simulink model "cl"  (Simulink 6.3)
settings: Solver=ode1  StartTime=0.0  StopTime=tsim_max  FixedStep=delt  RelTol=1e-3
values from neighbouring files (symbols this model uses):
  g = lp(i,1)    [gpm.m]
undefined symbols (not defined in the file or in its folder): Aac_trac, Asn, att1_step_cmd, att2_step_cmd, att3_step_cmd, att_type, Bac_trac, Bsn, c_att, c_rate, c_vel, ca_rate, ca_vel, Cac_trac, cbinv_rate, cbinv_vel, command_time, cosa, Cpos, ctht, Cvelpos, Dac_trac, delt, fb_att, fc_att, fc_pos, fc_rate, fc_vel, ff_att, fi_att, fi_pos, fi_rate, fi_vel, gthrot_step_cmd, ideal_d_actuator, ideal_engine_actuator, integ_d_a, integ_d_b, integ_d_c, integ_d_d, integ_engine_a, integ_engine_b, integ_engine_c, integ_engine_d, integ_gust_a, integ_gust_b, integ_gust_c, integ_gust_d, integ_MACH_att_a, integ_MACH_att_b, integ_MACH_att_c, integ_MACH_att_d, integ_MACH_att_ff_a, integ_MACH_att_ff_b, integ_MACH_att_ff_c, integ_MACH_att_ff_d, integ_MACH_pos_a, integ_MACH_pos_b, integ_MACH_pos_c, integ_MACH_pos_d ... (+53)
libraries: simulink x22
settings Model: LastModifiedBy=E704491  BufferReuse=off
settings DataIOCC: InitialState=[]  LoadInitialState=on
settings OptimizationCC: InlineParams=on  BufferReuse=off
settings DebuggingCC: AlgebraicLoopMsg=none

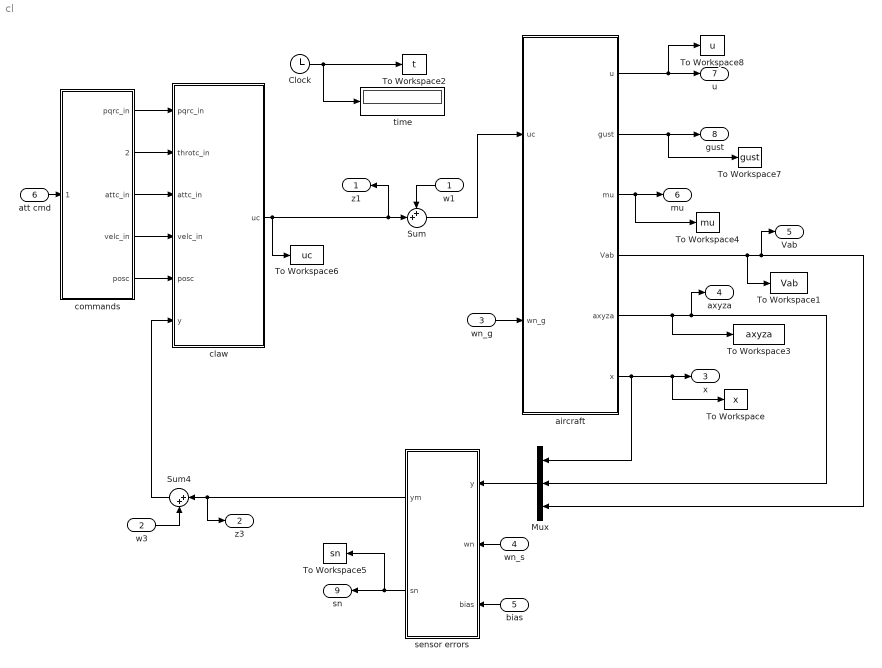
== system cl ==
  w1 : Inport  Orientation=left  PortDimensions=num_u
  w3 : Inport  Port=2  PortDimensions=num_y
  wn_g : Inport  Port=3  PortDimensions=3
  wn_s : Inport  Orientation=left  Port=4  PortDimensions=num_y
  bias : Inport  Orientation=left  Port=5  PortDimensions=num_y
  att cmd : Inport  Port=6
  Clock : Clock
      settings: Decimation=10
  Mux : Mux  Orientation=left  Inputs=3
  Sum : Sum  Inputs=++|
  Sum4 : Sum  Orientation=left  Inputs=|++
  To Workspace : ToWorkspace  VariableName=x  SampleTime=-1  SaveFormat=Array
  To Workspace1 : ToWorkspace  VariableName=Vab  SampleTime=-1  SaveFormat=Array
  To Workspace2 : ToWorkspace  VariableName=t  SampleTime=-1  SaveFormat=Array
  To Workspace3 : ToWorkspace  VariableName=axyza  SampleTime=-1  SaveFormat=Array
  To Workspace4 : ToWorkspace  VariableName=mu  SampleTime=-1  SaveFormat=Array
  To Workspace5 : ToWorkspace  VariableName=sn  SampleTime=-1  SaveFormat=Array
  To Workspace6 : ToWorkspace  VariableName=uc  SampleTime=-1  SaveFormat=Array
  To Workspace7 : ToWorkspace  VariableName=gust  SampleTime=-1  SaveFormat=Array
  To Workspace8 : ToWorkspace  VariableName=u  SampleTime=-1  SaveFormat=Array
  aircraft : Subsystem
  claw : Subsystem
  commands : Subsystem
  sensor errors : Subsystem  Orientation=left
  time : Display
  z1 : Outport  Orientation=left
  z3 : Outport  Port=2
  x : Outport  Port=3
  axyza : Outport  Port=4
  Vab : Outport  Port=5
  mu : Outport  Port=6
  u : Outport  Port=7
  gust : Outport  Port=8
  sn : Outport  Orientation=left  Port=9
  wires:
  claw/1(uc) -> Sum/2, z1/1, To Workspace6/1
  Clock/1 -> To Workspace2/1, time/1
  wn_s/1 -> sensor errors/2(wn)
  sensor errors/2(sn) -> sn/1, To Workspace5/1
  bias/1 -> sensor errors/3(bias)
  w1/1 -> Sum/1
  sensor errors/1(ym) -> Sum4/1, z3/1
  Sum4/1 -> claw/6(y)
  w3/1 -> Sum4/2
  aircraft/6(x) -> x/1, To Workspace/1, Mux/1
  aircraft/1(u) -> u/1, To Workspace8/1
  aircraft/4(Vab) -> To Workspace1/1, Vab/1, Mux/3
  Sum/1 -> aircraft/1(uc)
  wn_g/1 -> aircraft/2(wn_g)
  aircraft/2(gust) -> gust/1, To Workspace7/1
  commands/4(velc_in) -> claw/4(velc_in)
  aircraft/5(axyza) -> axyza/1, Mux/2, To Workspace3/1
  commands/5(posc) -> claw/5(posc)
  commands/2(throtc_in) -> claw/2(throtc_in)
  commands/3(attc_in) -> claw/3(attc_in)
  att cmd/1 -> commands/1(att cmd)
  Mux/1 -> sensor errors/1(y)
  aircraft/3(mu) -> mu/1, To Workspace4/1
  commands/1(pqrc_in) -> claw/1(pqrc_in)

== system cl/aircraft ==
  uc : Inport
  wn_g : Inport  Port=2
  actuators : Subsystem
  aircraft : Subsystem
  gust model : Subsystem
  u : Outport
  gust : Outport  Port=2
  mu : Outport  Port=3
  Vab : Outport  Port=4
  axyza : Outport  Port=5
  x : Outport  Port=6
  wires:
  aircraft/1(x) -> x/1
  aircraft/3(Vab) -> Vab/1
  wn_g/1 -> gust model/1(wn)
  gust model/1(gust) -> aircraft/2(gust), gust/1
  uc/1 -> actuators/1(uc)
  actuators/1(u) -> aircraft/1(u), u/1
  aircraft/2(axyza) -> axyza/1
  aircraft/4(mu) -> mu/1

== system cl/claw ==
  pqrc_in : Inport
  throtc_in : Inport  Port=2
  attc_in : Inport  Port=3
  velc_in : Inport  Port=4
  posc : Inport  Port=5
  y : Inport  Port=6
  MACH : Subsystem
  Mux : Mux  Inputs=2
  Mux1 : Mux  Inputs=5
  uc : Outport
  wires:
  attc_in/1 -> Mux1/3
  velc_in/1 -> Mux1/4
  Mux1/1 -> MACH/1(cmd)
  posc/1 -> Mux1/5
  y/1 -> MACH/2(y)
  MACH/1(d cmd) -> Mux/1
  MACH/2(throttle cmd) -> Mux/2
  Mux/1 -> uc/1
  throtc_in/1 -> Mux1/2
  pqrc_in/1 -> Mux1/1

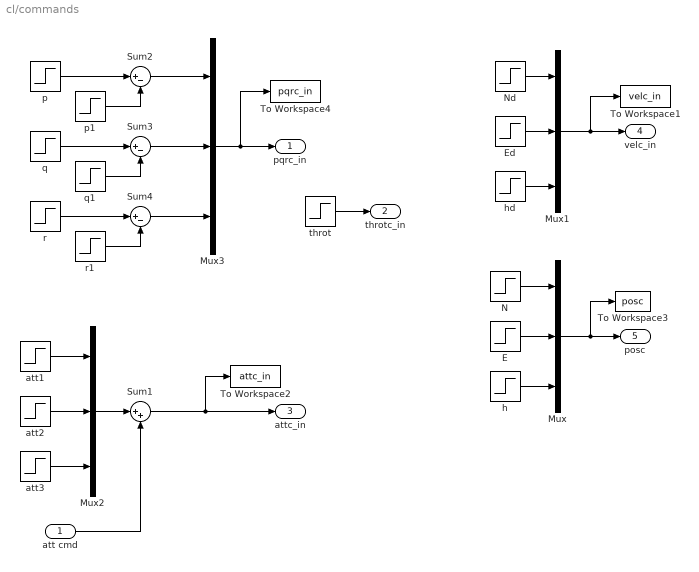
== system cl/commands ==
  att cmd : Inport  PortDimensions=3
  E : Step  Time=command_time  After=pos2_step_cmd  SampleTime=0
  Ed : Step  Time=command_time  After=vel2_step_cmd  SampleTime=0
  Mux{,1..3} (4 alike) : Mux  Inputs=3
  N : Step  Time=command_time  After=pos1_step_cmd  SampleTime=0
  Nd : Step  Time=command_time  After=vel1_step_cmd  SampleTime=0
  Sum1 : Sum  Inputs=|++
  Sum2 : Sum  Inputs=|+-
  Sum3 : Sum  Inputs=|+-
  Sum4 : Sum  Inputs=|+-
  To Workspace1 : ToWorkspace  VariableName=velc_in  SampleTime=-1  SaveFormat=Array
  To Workspace2 : ToWorkspace  VariableName=attc_in  SampleTime=-1  SaveFormat=Array
  To Workspace3 : ToWorkspace  VariableName=posc  SampleTime=-1  SaveFormat=Array
  To Workspace4 : ToWorkspace  VariableName=pqrc_in  SampleTime=-1  SaveFormat=Array
  att1 : Step  Time=command_time  After=att1_step_cmd  SampleTime=0
  att2 : Step  Time=command_time  After=att2_step_cmd  SampleTime=0
  att3 : Step  Time=command_time  After=att3_step_cmd  SampleTime=0
  h : Step  Time=command_time  After=pos3_step_cmd  SampleTime=0
  hd : Step  Time=command_time  After=vel3_step_cmd  SampleTime=0
  p : Step  Time=command_time  After=rate1_step_cmd  SampleTime=0
  p1 : Step  Time=command_time + pulse_width  After=rate1_step_cmd  SampleTime=0
  q : Step  Time=command_time  After=rate2_step_cmd  SampleTime=0
  q1 : Step  Time=command_time + pulse_width  After=rate2_step_cmd  SampleTime=0
  r : Step  Time=command_time  After=rate3_step_cmd  SampleTime=0
  r1 : Step  Time=command_time + pulse_width  After=rate3_step_cmd  SampleTime=0
  throt : Step  Time=command_time  After=gthrot_step_cmd  SampleTime=0
  pqrc_in : Outport
  throtc_in : Outport  Port=2
  attc_in : Outport  Port=3
  velc_in : Outport  Port=4
  posc : Outport  Port=5
  wires:
  h/1 -> Mux/3
  Nd/1 -> Mux1/1
  throt/1 -> throtc_in/1
  att2/1 -> Mux2/2
  att cmd/1 -> Sum1/2
  Mux/1 -> To Workspace3/1, posc/1
  Mux1/1 -> velc_in/1, To Workspace1/1
  att1/1 -> Mux2/1
  att3/1 -> Mux2/3
  Sum1/1 -> attc_in/1, To Workspace2/1
  Mux2/1 -> Sum1/1
  Mux3/1 -> pqrc_in/1, To Workspace4/1
  Sum2/1 -> Mux3/1
  p/1 -> Sum2/1
  Sum3/1 -> Mux3/2
  q/1 -> Sum3/1
  r/1 -> Sum4/1
  Sum4/1 -> Mux3/3
  p1/1 -> Sum2/2
  q1/1 -> Sum3/2
  r1/1 -> Sum4/2
  Ed/1 -> Mux1/2
  hd/1 -> Mux1/3
  N/1 -> Mux/1
  E/1 -> Mux/2

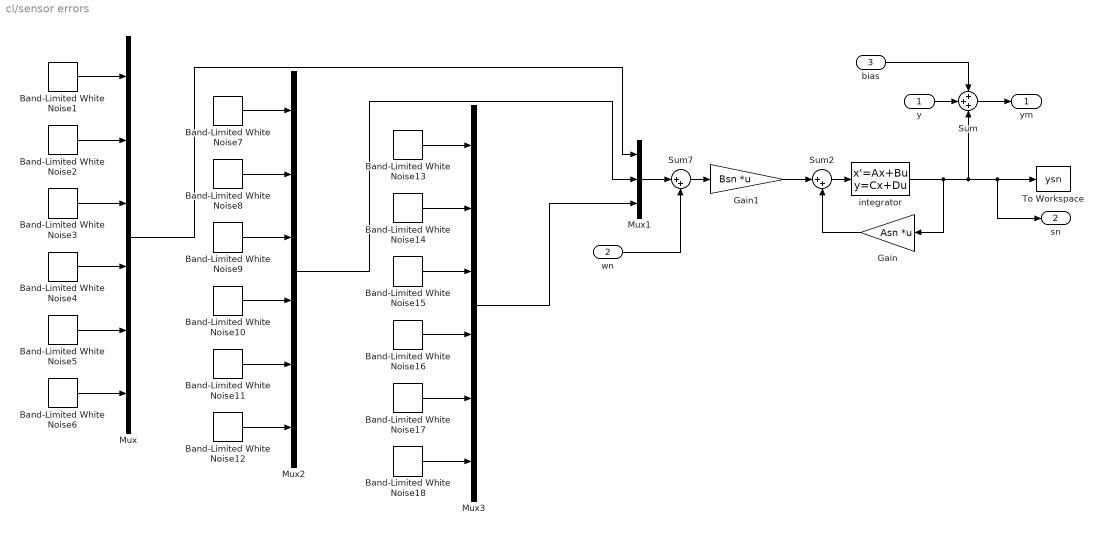
== system cl/sensor errors ==
  y : Inport
  wn : Inport  Port=2
  bias : Inport  Port=3
  Band-Limited White Noise1 : simulink/Sources/Band-Limited White Noise  Cov=1  Ts=delt  seed=sn_seed(1)
  Band-Limited White Noise10 : simulink/Sources/Band-Limited White Noise  Cov=1  Ts=delt  seed=sn_seed(10)
  Band-Limited White Noise11 : simulink/Sources/Band-Limited White Noise  Cov=1  Ts=delt  seed=sn_seed(11)
  Band-Limited White Noise12 : simulink/Sources/Band-Limited White Noise  Cov=1  Ts=delt  seed=sn_seed(12)
  Band-Limited White Noise13 : simulink/Sources/Band-Limited White Noise  Cov=1  Ts=delt  seed=sn_seed(13)
  Band-Limited White Noise14 : simulink/Sources/Band-Limited White Noise  Cov=1  Ts=delt  seed=sn_seed(14)
  Band-Limited White Noise15 : simulink/Sources/Band-Limited White Noise  Cov=1  Ts=delt  seed=sn_seed(15)
  Band-Limited White Noise16 : simulink/Sources/Band-Limited White Noise  Cov=1  Ts=delt  seed=sn_seed(16)
  Band-Limited White Noise17 : simulink/Sources/Band-Limited White Noise  Cov=1  Ts=delt  seed=sn_seed(17)
  Band-Limited White Noise18 : simulink/Sources/Band-Limited White Noise  Cov=1  Ts=delt  seed=sn_seed(18)
  Band-Limited White Noise2 : simulink/Sources/Band-Limited White Noise  Cov=1  Ts=delt  seed=sn_seed(2)
  Band-Limited White Noise3 : simulink/Sources/Band-Limited White Noise  Cov=1  Ts=delt  seed=sn_seed(3)
  Band-Limited White Noise4 : simulink/Sources/Band-Limited White Noise  Cov=1  Ts=delt  seed=sn_seed(4)
  Band-Limited White Noise5 : simulink/Sources/Band-Limited White Noise  Cov=1  Ts=delt  seed=sn_seed(5)
  Band-Limited White Noise6 : simulink/Sources/Band-Limited White Noise  Cov=1  Ts=delt  seed=sn_seed(6)
  Band-Limited White Noise7 : simulink/Sources/Band-Limited White Noise  Cov=1  Ts=delt  seed=sn_seed(7)
  Band-Limited White Noise8 : simulink/Sources/Band-Limited White Noise  Cov=1  Ts=delt  seed=sn_seed(8)
  Band-Limited White Noise9 : simulink/Sources/Band-Limited White Noise  Cov=1  Ts=delt  seed=sn_seed(9)
  Gain : Gain  Orientation=left  Gain=Asn  Multiplication=Matrix(K*u)
  Gain1 : Gain  Gain=Bsn  Multiplication=Matrix(K*u)
  Mux : Mux  Inputs=6
  Mux1 : Mux  Inputs=3
  Mux2 : Mux  Inputs=6
  Mux3 : Mux  Inputs=6
  Sum : Sum  Inputs=+++
  Sum2 : Sum  Inputs=|++
  Sum7 : Sum  Inputs=|++
  To Workspace : ToWorkspace  VariableName=ysn  SampleTime=-1  SaveFormat=Array
  integrator : StateSpace  A=integ_sn_a  B=integ_sn_b  C=integ_sn_c  D=integ_sn_d
  ym : Outport
  sn : Outport  Port=2
  wires:
  y/1 -> Sum/2
  Sum/1 -> ym/1
  Sum2/1 -> integrator/1
  Gain/1 -> Sum2/2
  integrator/1 -> Gain/1, Sum/3, To Workspace/1, sn/1
  Gain1/1 -> Sum2/1
  Sum7/1 -> Gain1/1
  Band-Limited White Noise4/1 -> Mux/4
  bias/1 -> Sum/1
  Band-Limited White Noise5/1 -> Mux/5
  Band-Limited White Noise6/1 -> Mux/6
  wn/1 -> Sum7/2
  Band-Limited White Noise1/1 -> Mux/1
  Band-Limited White Noise2/1 -> Mux/2
  Band-Limited White Noise3/1 -> Mux/3
  Mux1/1 -> Sum7/1
  Band-Limited White Noise10/1 -> Mux2/4
  Band-Limited White Noise11/1 -> Mux2/5
  Band-Limited White Noise12/1 -> Mux2/6
  Band-Limited White Noise7/1 -> Mux2/1
  Band-Limited White Noise8/1 -> Mux2/2
  Band-Limited White Noise9/1 -> Mux2/3
  Band-Limited White Noise16/1 -> Mux3/4
  Band-Limited White Noise17/1 -> Mux3/5
  Band-Limited White Noise18/1 -> Mux3/6
  Band-Limited White Noise13/1 -> Mux3/1
  Band-Limited White Noise14/1 -> Mux3/2
  Band-Limited White Noise15/1 -> Mux3/3
  Mux/1 -> Mux1/1
  Mux2/1 -> Mux1/2
  Mux3/1 -> Mux1/3

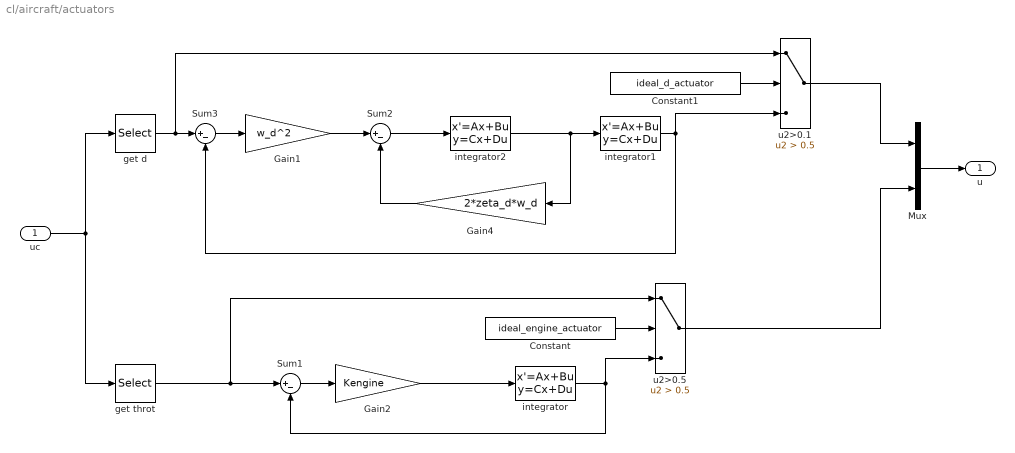
== system cl/aircraft/actuators ==
  uc : Inport
  Constant : Constant  Value=ideal_engine_actuator
  Constant1 : Constant  Value=ideal_d_actuator
  Gain1 : Gain  Gain=w_d^2
  Gain2 : Gain  Gain=Kengine
  Gain4 : Gain  Orientation=left  Gain=2*zeta_d*w_d
  Mux : Mux  Inputs=2
  Sum1 : Sum  Inputs=|+-
  Sum2 : Sum  Inputs=|+-
  Sum3 : Sum  Inputs=|+-
  get d : Selector  Elements=iu_d  InputPortWidth=num_u
  get throt : Selector  Elements=iu_throt  InputPortWidth=num_u
  integrator : StateSpace  A=integ_engine_a  B=integ_engine_b  C=integ_engine_c  D=integ_engine_d
  integrator1 : StateSpace  A=integ_d_a  B=integ_d_b  C=integ_d_c  D=integ_d_d
  integrator2 : StateSpace  A=integ_d_a  B=integ_d_b  C=integ_d_c  D=integ_d_d
  u2>0.1 : Switch  Criteria=u2 > Threshold  Threshold=0.5
  u2>0.5 : Switch  Criteria=u2 > Threshold  Threshold=0.5
  u : Outport
  wires:
  Gain2/1 -> integrator/1
  Sum1/1 -> Gain2/1
  integrator1/1 -> Sum3/2, u2>0.1/3
  integrator2/1 -> Gain4/1, integrator1/1
  Sum2/1 -> integrator2/1
  Gain4/1 -> Sum2/2
  Gain1/1 -> Sum2/1
  integrator/1 -> Sum1/2, u2>0.5/3
  get throt/1 -> Sum1/1, u2>0.5/1
  uc/1 -> get d/1, get throt/1
  Sum3/1 -> Gain1/1
  Constant/1 -> u2>0.5/2
  Constant1/1 -> u2>0.1/2
  get d/1 -> Sum3/1, u2>0.1/1
  Mux/1 -> u/1
  u2>0.1/1 -> Mux/1
  u2>0.5/1 -> Mux/2

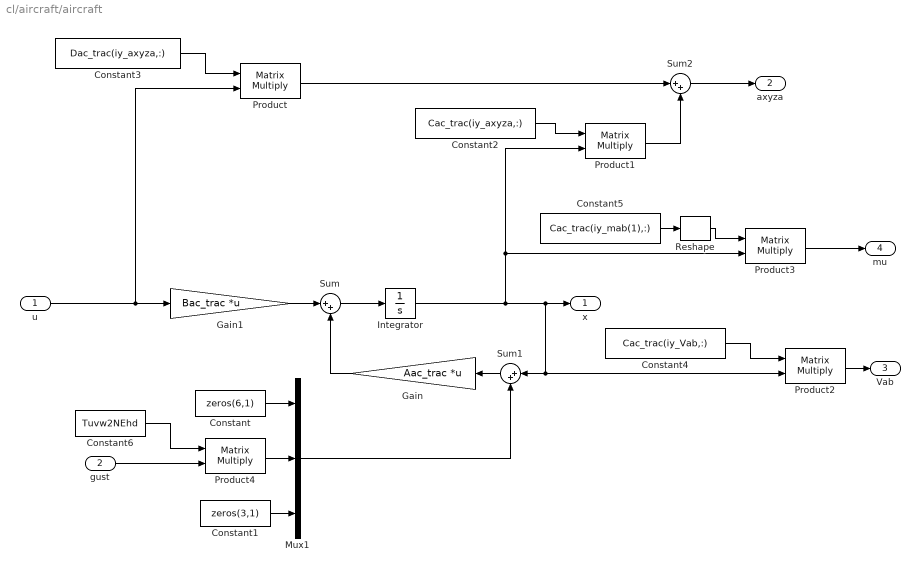
== system cl/aircraft/aircraft ==
  u : Inport
  gust : Inport  Port=2
  Constant : Constant  Value=zeros(6,1)
  Constant1 : Constant  Value=zeros(3,1)
  Constant2 : Constant  Value=Cac_trac(iy_axyza,:)
  Constant3 : Constant  Value=Dac_trac(iy_axyza,:)
  Constant4 : Constant  Value=Cac_trac(iy_Vab,:)
  Constant5 : Constant  Value=Cac_trac(iy_mab(1),:)
  Constant6 : Constant  Value=Tuvw2NEhd
  Gain : Gain  Orientation=left  Gain=Aac_trac  Multiplication=Matrix(K*u)
  Gain1 : Gain  Gain=Bac_trac  Multiplication=Matrix(K*u)
  Integrator : Integrator
  Mux1 : Mux  Inputs=3
  Product{,1..4} (5 alike) : Product  Multiplication=Matrix(*)  RndMeth=Zero
  Reshape : simulink/Math Operations/Reshape  OutputDimensionality=Row vector  OutputDimensions=[1,1]
  Sum : Sum  Inputs=|++
  Sum1 : Sum  Orientation=left  Inputs=|++
  Sum2 : Sum  Inputs=|++
  x : Outport
  axyza : Outport  Port=2
  Vab : Outport  Port=3
  mu : Outport  Port=4
  wires:
  Integrator/1 -> x/1, Sum1/1, Product2/2, Product1/2, Product3/2
  Sum/1 -> Integrator/1
  Gain1/1 -> Sum/1
  Gain/1 -> Sum/2
  u/1 -> Gain1/1, Product/2
  Constant1/1 -> Mux1/3
  Sum1/1 -> Gain/1
  Mux1/1 -> Sum1/2
  Constant/1 -> Mux1/1
  Constant3/1 -> Product/1
  Constant2/1 -> Product1/1
  Product1/1 -> Sum2/2
  Product/1 -> Sum2/1
  Sum2/1 -> axyza/1
  Constant4/1 -> Product2/1
  Product2/1 -> Vab/1
  Constant5/1 -> Reshape/1
  Product3/1 -> mu/1
  Reshape/1 -> Product3/1
  Constant6/1 -> Product4/1
  Product4/1 -> Mux1/2
  gust/1 -> Product4/2

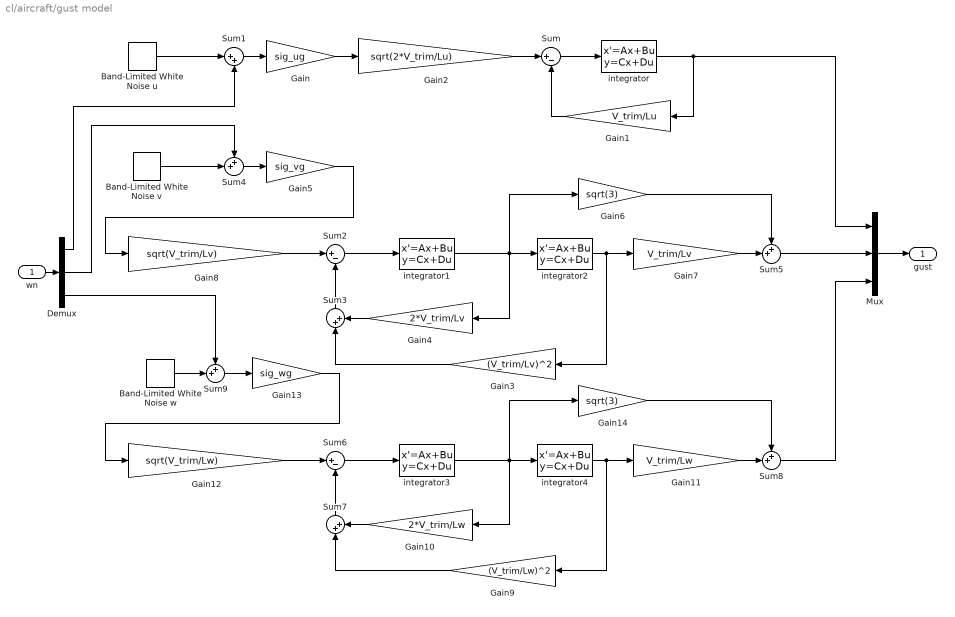
== system cl/aircraft/gust model ==
  wn : Inport
  Band-Limited White Noise u : simulink/Sources/Band-Limited White Noise  Cov=[1]  Ts=delt  seed=[ 82141 ]
  Band-Limited White Noise v : simulink/Sources/Band-Limited White Noise  Cov=[1]  Ts=delt  seed=[ 44470 ]
  Band-Limited White Noise w : simulink/Sources/Band-Limited White Noise  Cov=[1]  Ts=delt  seed=[ 93181 ]
  Demux : Demux  Outputs=3
  Gain : Gain  Gain=sig_ug
  Gain1 : Gain  Orientation=left  Gain=V_trim/Lu
  Gain10 : Gain  Orientation=left  Gain=2*V_trim/Lw
  Gain11 : Gain  Gain=V_trim/Lw
  Gain12 : Gain  Gain=sqrt(V_trim/Lw)
  Gain13 : Gain  Gain=sig_wg
  Gain14 : Gain  Gain=sqrt(3)
  Gain2 : Gain  Gain=sqrt(2*V_trim/Lu)
  Gain3 : Gain  Orientation=left  Gain=(V_trim/Lv)^2
  Gain4 : Gain  Orientation=left  Gain=2*V_trim/Lv
  Gain5 : Gain  Gain=sig_vg
  Gain6 : Gain  Gain=sqrt(3)
  Gain7 : Gain  Gain=V_trim/Lv
  Gain8 : Gain  Gain=sqrt(V_trim/Lv)
  Gain9 : Gain  Orientation=left  Gain=(V_trim/Lw)^2
  Mux : Mux  Inputs=3
  Sum : Sum  Inputs=|+-
  Sum1 : Sum  Inputs=|++
  Sum2 : Sum  Inputs=|+-
  Sum3 : Sum  Orientation=up  Inputs=|++
  Sum{4..5,8..9} (4 alike) : Sum  Inputs=++|
  Sum6 : Sum  Inputs=|+-
  Sum7 : Sum  Orientation=up  Inputs=|++
  integrator{,1..4} (5 alike) : StateSpace  A=integ_gust_a  B=integ_gust_b  C=integ_gust_c  D=integ_gust_d
  gust : Outport
  wires:
  integrator/1 -> Gain1/1, Mux/1
  Gain1/1 -> Sum/2
  Sum/1 -> integrator/1
  Gain/1 -> Gain2/1
  Gain2/1 -> Sum/1
  Sum1/1 -> Gain/1
  Band-Limited White Noise u/1 -> Sum1/1
  integrator2/1 -> Gain3/1, Gain7/1
  integrator1/1 -> Gain4/1, Gain6/1, integrator2/1
  Sum2/1 -> integrator1/1
  Sum3/1 -> Sum2/2
  Gain4/1 -> Sum3/2
  Gain3/1 -> Sum3/1
  Sum4/1 -> Gain5/1
  Band-Limited White Noise v/1 -> Sum4/2
  Sum5/1 -> Mux/2
  Gain6/1 -> Sum5/1
  Gain7/1 -> Sum5/2
  Gain8/1 -> Sum2/1
  Gain5/1 -> Gain8/1
  Mux/1 -> gust/1
  integrator4/1 -> Gain9/1, Gain11/1
  integrator3/1 -> Gain10/1, integrator4/1, Gain14/1
  Sum6/1 -> integrator3/1
  Sum7/1 -> Sum6/2
  Gain10/1 -> Sum7/2
  Gain9/1 -> Sum7/1
  Sum8/1 -> Mux/3
  Gain14/1 -> Sum8/1
  Gain11/1 -> Sum8/2
  Gain12/1 -> Sum6/1
  Gain13/1 -> Gain12/1
  Sum9/1 -> Gain13/1
  Band-Limited White Noise w/1 -> Sum9/2
  wn/1 -> Demux/1
  Demux/1 -> Sum1/2
  Demux/2 -> Sum4/1
  Demux/3 -> Sum9/1

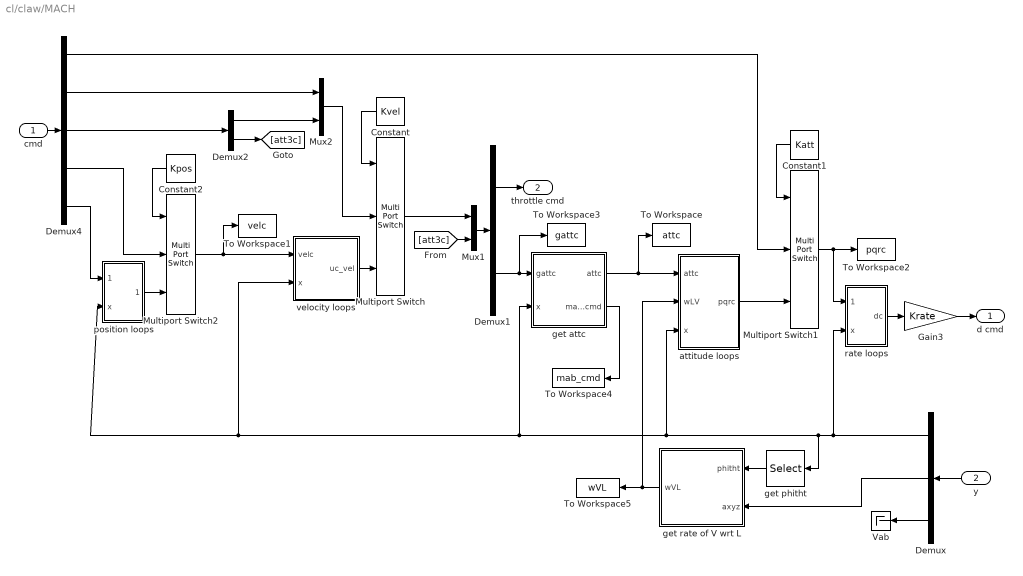
== system cl/claw/MACH ==
  cmd : Inport
  y : Inport  Orientation=left  Port=2
  Constant : Constant  Orientation=left  Value=Kvel
  Constant1 : Constant  Orientation=left  Value=Katt
  Constant2 : Constant  Orientation=left  Value=Kpos
  Demux : Demux  Orientation=left  Outputs=[ 12 3 3 ]
  Demux1 : Demux  Outputs=[ 1 3 ]
  Demux2 : Demux  Outputs=[ 2 1 ]
  Demux4 : Demux  Outputs=[ 3 1 3 3 3 ]
  Gain3 : Gain  Gain=Krate
  Multiport Switch : MultiPortSwitch  Inputs=2  zeroidx=on
  Multiport Switch1 : MultiPortSwitch  Inputs=2  zeroidx=on
  Multiport Switch2 : MultiPortSwitch  Inputs=2  zeroidx=on
  Mux1 : Mux  Inputs=2
  Mux2 : Mux  Inputs=2
  To Workspace : ToWorkspace  VariableName=attc  SampleTime=-1  SaveFormat=Array
  To Workspace1 : ToWorkspace  VariableName=velc  SampleTime=-1  SaveFormat=Array
  To Workspace2 : ToWorkspace  VariableName=pqrc  SampleTime=-1  SaveFormat=Array
  To Workspace3 : ToWorkspace  VariableName=gattc  SampleTime=-1  SaveFormat=Array
  To Workspace4 : ToWorkspace  VariableName=mab_cmd  SampleTime=-1  SaveFormat=Array
  To Workspace5 : ToWorkspace  VariableName=wVL  SampleTime=-1  SaveFormat=Array
  Vab : Terminator
  attitude loops : Subsystem
  get attc : Subsystem
  get phitht : Selector  Orientation=left  Elements=i_phitht  InputPortWidth=12
  get rate of V wrt L : Subsystem  Orientation=left
  position loops : Subsystem
  rate loops : Subsystem
  velocity loops : Subsystem
  d cmd : Outport
  throttle cmd : Outport  Port=2
  wires:
  velocity loops/1(uc_vel) -> Multiport Switch/3
  Constant/1 -> Multiport Switch/1
  Demux4/5 -> position loops/1(posc)
  Mux2/1 -> Multiport Switch/2
  get rate of V wrt L/1(wVL) -> attitude loops/2(wLV), To Workspace5/1
  get attc/2(mab_cmd) -> To Workspace4/1
  get attc/1(attc) -> To Workspace/1, attitude loops/1(attc)
  Demux1/2 -> get attc/1(gattc), To Workspace3/1
  Demux1/1 -> throttle cmd/1
  Gain3/1 -> d cmd/1
  Multiport Switch1/1 -> rate loops/1(pqrc), To Workspace2/1
  Multiport Switch2/1 -> velocity loops/1(velc), To Workspace1/1
  rate loops/1(dc) -> Gain3/1
  y/1 -> Demux/1
  attitude loops/1(pqrc) -> Multiport Switch1/3
  Demux/1 -> rate loops/2(x), get attc/2(x), velocity loops/2(x), position loops/2(x), attitude loops/3(x), get phitht/1
  Demux4/2 -> Mux2/1
  Demux4/4 -> Multiport Switch2/2
  Demux4/3 -> Demux2/1
  Demux2/1 -> Mux2/2
  Multiport Switch/1 -> Mux1/1
  Mux1/1 -> Demux1/1
  Demux/3 -> Vab/1
  Demux/2 -> get rate of V wrt L/2(axyz)
  get phitht/1 -> get rate of V wrt L/1(phitht)
  Constant1/1 -> Multiport Switch1/1
  cmd/1 -> Demux4/1
  Demux4/1 -> Multiport Switch1/2
  Demux2/2 -> [att3c]
  [att3c] -> Mux1/2
  position loops/1(velc) -> Multiport Switch2/3
  Constant2/1 -> Multiport Switch2/1

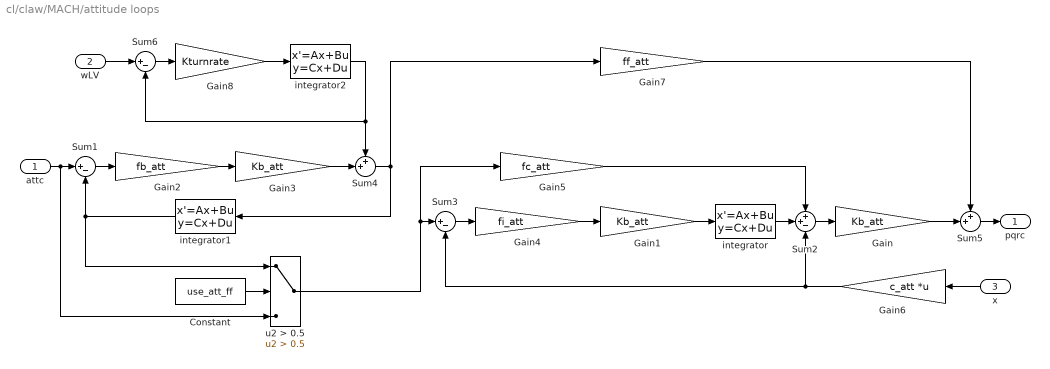
== system cl/claw/MACH/attitude loops ==
  attc : Inport
  wLV : Inport  Port=2
  x : Inport  Orientation=left  Port=3
  Constant : Constant  Value=use_att_ff
  Gain : Gain  Gain=Kb_att
  Gain1 : Gain  Gain=Kb_att
  Gain2 : Gain  Gain=fb_att
  Gain3 : Gain  Gain=Kb_att
  Gain4 : Gain  Gain=fi_att
  Gain5 : Gain  Gain=fc_att
  Gain6 : Gain  Orientation=left  Gain=c_att  Multiplication=Matrix(K*u)
  Gain7 : Gain  Gain=ff_att
  Gain8 : Gain  Gain=Kturnrate
  Sum1 : Sum  Inputs=|+-
  Sum2 : Sum  Inputs=++-
  Sum3 : Sum  Inputs=|+-
  Sum4 : Sum  Inputs=++|
  Sum5 : Sum  Inputs=++|
  Sum6 : Sum  Inputs=|+-
  integrator : StateSpace  A=integ_MACH_att_a  B=integ_MACH_att_b  C=integ_MACH_att_c  D=integ_MACH_att_d
  integrator1 : StateSpace  Orientation=left  A=integ_MACH_att_ff_a  B=integ_MACH_att_ff_b  C=integ_MACH_att_ff_c  D=integ_MACH_att_ff_d
  integrator2 : StateSpace  A=integ_MACH_att_ff_a  B=integ_MACH_att_ff_b  C=integ_MACH_att_ff_c  D=integ_MACH_att_ff_d
  u2 > 0.5 : Switch  Criteria=u2 > Threshold  Threshold=0.5
  pqrc : Outport
  wires:
  Gain8/1 -> integrator2/1
  wLV/1 -> Sum6/1
  Sum6/1 -> Gain8/1
  integrator2/1 -> Sum6/2, Sum4/1
  Gain7/1 -> Sum5/1
  Sum5/1 -> pqrc/1
  Gain/1 -> Sum5/2
  Sum4/1 -> Gain7/1, integrator1/1
  Gain3/1 -> Sum4/2
  u2 > 0.5/1 -> Sum3/1, Gain5/1
  Constant/1 -> u2 > 0.5/2
  Gain2/1 -> Gain3/1
  Sum1/1 -> Gain2/1
  attc/1 -> u2 > 0.5/3, Sum1/1
  integrator1/1 -> u2 > 0.5/1, Sum1/2
  integrator/1 -> Sum2/2
  Gain6/1 -> Sum2/3, Sum3/2
  Sum3/1 -> Gain4/1
  Gain1/1 -> integrator/1
  Gain4/1 -> Gain1/1
  Gain5/1 -> Sum2/1
  Sum2/1 -> Gain/1
  x/1 -> Gain6/1

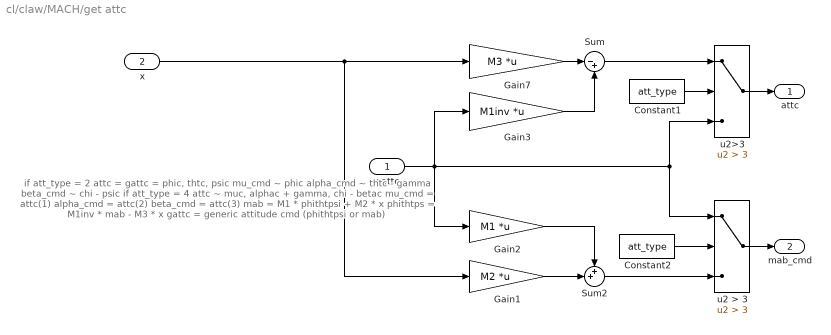
== system cl/claw/MACH/get attc ==
  note: if att_type = 2
      | attc = gattc = phic, thtc, psic
      | mu_cmd ~ phic
      | alpha_cmd ~ thtc - gamma
      | beta_cmd ~ chi - psic
      |
      | if att_type = 4
      | attc ~ muc, alphac + gamma, chi - betac
      | mu_cmd = attc(1)
      | alpha_cmd = attc(2)
      | beta_cmd = attc(3)
      |
      | mab = M1 * phithtpsi + M2 * x
      | phithtps = M1inv * mab - M3 * x
      |
      | gattc = generic attitude cmd (phithtpsi or mab)
  gattc : Inport
  x : Inport  Port=2
  Constant1 : Constant  Value=att_type
  Constant2 : Constant  Value=att_type
  Gain1 : Gain  Gain=M2  Multiplication=Matrix(K*u)
  Gain2 : Gain  Gain=M1  Multiplication=Matrix(K*u)
  Gain3 : Gain  Gain=M1inv  Multiplication=Matrix(K*u)
  Gain7 : Gain  Gain=M3  Multiplication=Matrix(K*u)
  Sum : Sum  Inputs=|-+
  Sum2 : Sum  Inputs=++|
  u2 > 3 : Switch  Criteria=u2 > Threshold  Threshold=3
  u2>3 : Switch  Criteria=u2 > Threshold  Threshold=3
  attc : Outport
  mab_cmd : Outport  Port=2
  wires:
  gattc/1 -> u2 > 3/1, u2>3/3, Gain2/1, Gain3/1
  x/1 -> Gain7/1, Gain1/1
  Constant1/1 -> u2>3/2
  u2>3/1 -> attc/1
  Sum/1 -> u2>3/1
  Constant2/1 -> u2 > 3/2
  u2 > 3/1 -> mab_cmd/1
  Sum2/1 -> u2 > 3/3
  Gain7/1 -> Sum/1
  Gain1/1 -> Sum2/2
  Gain2/1 -> Sum2/1
  Gain3/1 -> Sum/2

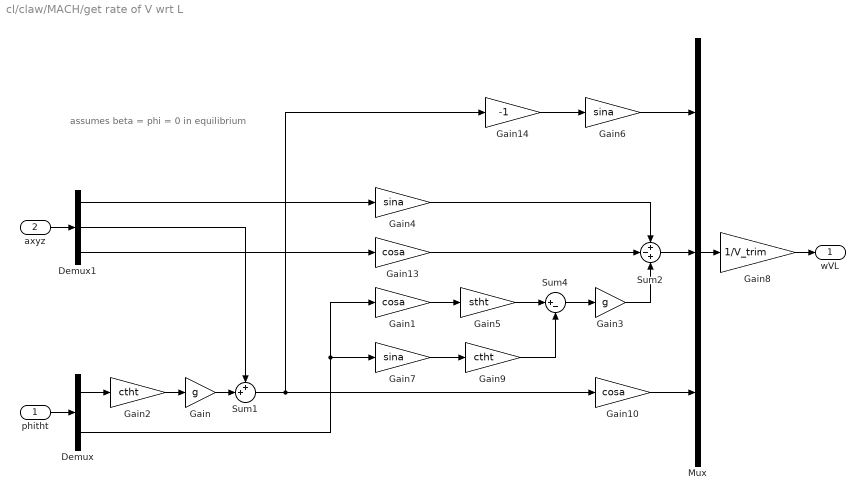
== system cl/claw/MACH/get rate of V wrt L ==
  note: assumes beta = phi = 0 in equilibrium
  phitht : Inport
  axyz : Inport  Port=2
  Demux : Demux  Outputs=2
  Demux1 : Demux  Outputs=3
  Gain : Gain  Gain=g
  Gain1 : Gain  Gain=cosa
  Gain10 : Gain  Gain=cosa
  Gain13 : Gain  Gain=cosa
  Gain14 : Gain  Gain=-1
  Gain2 : Gain  Gain=ctht
  Gain3 : Gain  Gain=g
  Gain4 : Gain  Gain=sina
  Gain5 : Gain  Gain=stht
  Gain6 : Gain  Gain=sina
  Gain7 : Gain  Gain=sina
  Gain8 : Gain  Gain=1/V_trim
  Gain9 : Gain  Gain=ctht
  Mux : Mux  Inputs=3
  Sum1 : Sum  Inputs=++|
  Sum2 : Sum  Inputs=+-+
  Sum4 : Sum  Inputs=|+-
  wVL : Outport
  wires:
  Gain8/1 -> wVL/1
  axyz/1 -> Demux1/1
  phitht/1 -> Demux/1
  Mux/1 -> Gain8/1
  Gain/1 -> Sum1/2
  Gain2/1 -> Gain/1
  Sum2/1 -> Mux/2
  Demux1/1 -> Gain4/1
  Demux1/2 -> Sum1/1
  Demux1/3 -> Gain13/1
  Demux/1 -> Gain2/1
  Demux/2 -> Gain1/1, Gain7/1
  Gain4/1 -> Sum2/1
  Gain1/1 -> Gain5/1
  Gain7/1 -> Gain9/1
  Gain6/1 -> Mux/1
  Gain10/1 -> Mux/3
  Sum4/1 -> Gain3/1
  Gain5/1 -> Sum4/1
  Gain9/1 -> Sum4/2
  Gain3/1 -> Sum2/3
  Gain13/1 -> Sum2/2
  Gain14/1 -> Gain6/1
  Sum1/1 -> Gain14/1, Gain10/1

== system cl/claw/MACH/position loops ==
  posc : Inport
  x : Inport  Orientation=left  Port=2
  Gain : Gain  Gain=Kb_pos
  Gain1 : Gain  Gain=Kb_pos
  Gain4 : Gain  Gain=fi_pos
  Gain5 : Gain  Gain=fc_pos
  Gain7 : Gain  Orientation=left  Gain=Cpos  Multiplication=Matrix(K*u)
  Sum2 : Sum  Inputs=++-
  Sum3 : Sum  Inputs=|+-
  integrator : StateSpace  A=integ_MACH_pos_a  B=integ_MACH_pos_b  C=integ_MACH_pos_c  D=integ_MACH_pos_d
  velc : Outport
  wires:
  integrator/1 -> Sum2/2
  posc/1 -> Sum3/1, Gain5/1
  Sum3/1 -> Gain4/1
  Gain1/1 -> integrator/1
  Gain4/1 -> Gain1/1
  Gain5/1 -> Sum2/1
  Sum2/1 -> Gain/1
  Gain/1 -> velc/1
  x/1 -> Gain7/1
  Gain7/1 -> Sum2/3, Sum3/2

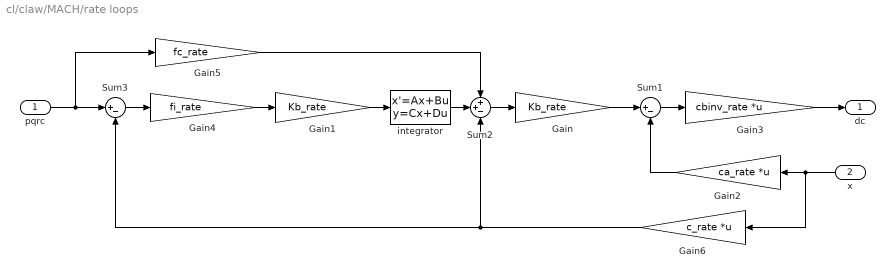
== system cl/claw/MACH/rate loops ==
  pqrc : Inport
  x : Inport  Orientation=left  Port=2
  Gain : Gain  Gain=Kb_rate
  Gain1 : Gain  Gain=Kb_rate
  Gain2 : Gain  Orientation=left  Gain=ca_rate  Multiplication=Matrix(K*u)
  Gain3 : Gain  Gain=cbinv_rate  Multiplication=Matrix(K*u)
  Gain4 : Gain  Gain=fi_rate
  Gain5 : Gain  Gain=fc_rate
  Gain6 : Gain  Orientation=left  Gain=c_rate  Multiplication=Matrix(K*u)
  Sum1 : Sum  Inputs=|+-
  Sum2 : Sum  Inputs=++-
  Sum3 : Sum  Inputs=|+-
  integrator : StateSpace  A=integ_MACH_rate_a  B=integ_MACH_rate_b  C=integ_MACH_rate_c  D=integ_MACH_rate_d
  dc : Outport
  wires:
  integrator/1 -> Sum2/2
  Gain3/1 -> dc/1
  pqrc/1 -> Sum3/1, Gain5/1
  Gain6/1 -> Sum2/3, Sum3/2
  Sum3/1 -> Gain4/1
  Gain1/1 -> integrator/1
  Gain4/1 -> Gain1/1
  Gain5/1 -> Sum2/1
  Sum2/1 -> Gain/1
  Gain/1 -> Sum1/1
  x/1 -> Gain2/1, Gain6/1
  Gain2/1 -> Sum1/2
  Sum1/1 -> Gain3/1

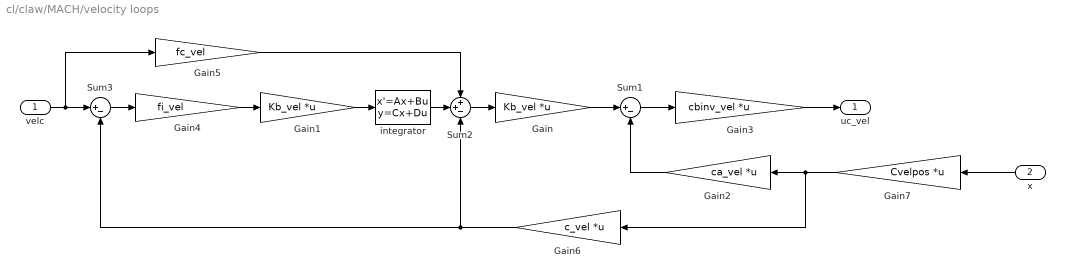
== system cl/claw/MACH/velocity loops ==
  velc : Inport
  x : Inport  Orientation=left  Port=2
  Gain : Gain  Gain=Kb_vel  Multiplication=Matrix(K*u)
  Gain1 : Gain  Gain=Kb_vel  Multiplication=Matrix(K*u)
  Gain2 : Gain  Orientation=left  Gain=ca_vel  Multiplication=Matrix(K*u)
  Gain3 : Gain  Gain=cbinv_vel  Multiplication=Matrix(K*u)
  Gain4 : Gain  Gain=fi_vel
  Gain5 : Gain  Gain=fc_vel
  Gain6 : Gain  Orientation=left  Gain=c_vel  Multiplication=Matrix(K*u)
  Gain7 : Gain  Orientation=left  Gain=Cvelpos  Multiplication=Matrix(K*u)
  Sum1 : Sum  Inputs=|+-
  Sum2 : Sum  Inputs=++-
  Sum3 : Sum  Inputs=|+-
  integrator : StateSpace  A=integ_MACH_vel_a  B=integ_MACH_vel_b  C=integ_MACH_vel_c  D=integ_MACH_vel_d
  uc_vel : Outport
  wires:
  integrator/1 -> Sum2/2
  Gain7/1 -> Gain2/1, Gain6/1
  Gain3/1 -> uc_vel/1
  velc/1 -> Sum3/1, Gain5/1
  Gain6/1 -> Sum2/3, Sum3/2
  Sum3/1 -> Gain4/1
  Gain1/1 -> integrator/1
  Gain4/1 -> Gain1/1
  Gain5/1 -> Sum2/1
  Sum2/1 -> Gain/1
  Gain/1 -> Sum1/1
  x/1 -> Gain7/1
  Gain2/1 -> Sum1/2
  Sum1/1 -> Gain3/1
